simulink model "pulse_heating_official_spine_v04"  (R2025b)
settings: Solver=VariableStepAuto  StartTime=0.0  StopTime=0.25  RelTol=1e-3
PreLoadFcn:
  | addpath('C:\Users\ADMIN\Documents\MATLAB\Examples\R2025b\simscapeelectrical\BatteryThermalManagementExample');
  | addpath('C:\Users\ADMIN\Documents\MATLAB\Examples\R2025b\mcb\SIUnitsExample');
  | addpath('C:\Users\ADMIN\Documents\MATLAB\Examples\R2025b\simscapeelectrical\PMSMDriveThermalExample');
  | load_system('PMSMDriveThermal');
  | set_param('PMSMDriveThermal','SimscapeLogType','none','SimscapeLogSimulationStatistics','off');
  | set_param('PMSMDriveThermal','Dirty','off');
InitFcn:
  | % === M4-02A: Clean parameter matching (MO theory PI) ===
  | addpath('C:\Users\ADMIN\Documents\MATLAB\Examples\R2025b\simscapeelectrical\BatteryThermalManagementExample');
  | addpath('C:\Users\ADMIN\Documents\MATLAB\Examples\R2025b\mcb\SIUnitsExample');
  | addpath('C:\Users\ADMIN\Documents\MATLAB\Examples\R2025b\simscapeelectrical\PMSMDriveThermalExample');
  | load_system('PMSMDriveThermal');
  | PMSMDriveThermalData;
  | mcb_pmsm_foc_qep_f28379d_SIUnit_data;
  | clearvars('all');
  | 
  | % --- Construct clean pmsm struct from PMSMDriveThermal ---
  | pmsm = struct();
  | pmsm.Rs = Rs; pmsm.Ld = Ld; pmsm.Lq = Lq; pmsm.p = N; pmsm.FluxPM = PM;
  | pmsm.J = J; pmsm.B = 2.6369e-6; pmsm.I_rated = Imax;
  | pmsm.Ke = PM*N; pmsm.Kt = 1.5*N*PM; pmsm.N_max = 60*fnom/N;
  | pmsm.PositionOffset = 0; pmsm.QEPSlits = 1000;
  | 
  | inverter.V_dc = 70; dataType = 'double';
  | pmsm.N_base = inverter.V_dc / (sqrt(3)*PM*N*2*pi/60);
  | pmsm.T_rated = 1.5*N*PM*Imax;
  | 
  | % --- Timing (PMSMDriveThermal semantics) ---
  | Ts = 2e-6; fsw = 2e3; fc = fsw*10; Tsc = 1/fc;
  | T_pwm = 1/fsw; PWM_frequency = fsw; Ts_simulink = Tsc;
  | Ts_motor = Tsc; Ts_speed = 10*Tsc; Ts_inverter = Tsc;
  | 
  | % --- PI gains via mcb.calcFOCGains (MO theory) ---
  | motor = pmsm; motor.Rs = pmsm.Rs + inverter.R_board;
  | PI_params = mcb.calcFOCGains(motor, Tsc, Ts_speed, SpdLPFltCoeff=0.01);
  | PI_params.delay_Currents = int32(1);
  | PI_params.delay_Position = int32(1);
  | 
  | BatteryThermalManagementInitialization;
  | ambient = 263.15; coolantTemp = 263.15;
  | cellT_ini = ambient*ones(1,Ns*Np); cellT_ini4 = ambient*ones(1,Ns4*Np4);
  | Ns_total = 3*Ns + Ns4; Np_total = Np;
  | R_pack = Ns_total * R0_mat(3,2) / Np_total;
  | I_base_A = AH * Np_total; V_pack_nom = Ns_total * 3.3;
  | 
  | % === M4-01 generalized Reference / Platform contract ===
  | % Values are traceable engineering/platform defaults, not device ratings.
  | ReferenceConfig_ID = 'M4-01-REF-PLATFORM-v02';
  | ReferenceConfig_Source = 'OFFICIAL+ENGINEERING_DEFAULT';
  | ReferenceConfig_Scope = 'generalized_system_integration';
  | HVPath_R = 0.01;
  | DCLink_C = 470e-6;
  | DCLink_V0 = 0;
  | RMS_Window_s = 20/fsw;
  | IGBT_Ron_ref = 1e-3;
  | IGBT_Vf_ref = 1.2;
  | 
  | % Encoder/reference topology provides the static mechanical boundary.
  | OpenLoop_Vabc_Scale = 1;
model workspace (MAT data in the model file):
  control_status_v4d2_partial_duty_code = 6
  diagnostic_frequency_Hz = 50
  drive_status_v4d2_partial_current_code = 6
  kpi_status_v4d2_partial_numeric_code = 6
  kpi_value_unknown = nan
  limit_factor_unknown_code = 99
  limit_margin_unknown_value = nan
  limit_status_v4c_code = 5
  pulse_command_status_code = 6
  pulse_duty_percent = 50
  pulse_id_amplitude_A = 40
  pulse_iq_amplitude_A = 0
  pulse_mode_code = 4
  pulse_phase_delay_s = 0
undefined symbols (not defined in the file or in its folder): DiscIntNeverNeededParam, f_losses, Flowrate_vec, Isc_losses, losses_oc, losses_sc, N, PM, Rs
libraries: fl_lib x38, nesl_utility x35, ee_lib x12, mcbcontrolslib x5, mcbeeMathTransformLib x3, slpidlib x2, mcbhdlpositiondecoderlib x1, eePwmGeneratorTwoLevel x1
(part 3 of 4)

== system pulse_heating_official_spine_v04/PMSMDriveThermal_Inverter_And_Motor/Three-phase inverter ==
  G : Inport
  Demux : Demux  Outputs=6
  IGBT A(H) : ee_lib/Semiconductors & Converters/IGBT (Ideal, Switching)  port_option=ee.enum.controlport.ps  Vf=0.8 V  Ron=0.001 Ohm  Goff=1e-5 S  Vth=0.5 V  diode_param=2  diode_Vf=0.8 V  diode_Ron=0.001 Ohm  diode_Goff=1e-5 S  diode_C=5e-8 F  diode_iRM=-235 A  diode_iF=300 A  diode_idot=-50 A/us  diode_trr_param=1  diode_trr_factor=3  diode_trr=15 us  diode_Qrr=1.5e+3 s*uA  ice_specify=off  ice_priority=None  ice=0 A  ice_nominal_specify=off  ice_nominal_value=1  ice_nominal_unit=A  vce_specify=off  vce_priority=None  vce=0 V  vce_nominal_specify=off  vce_nominal_value=1  vce_nominal_unit=V  vge_specify=off  vge_priority=None  vge=0 V  vge_nominal_specify=off  vge_nominal_value=1  vge_nominal_unit=V  thermal_loss_option=ee.enum.converters.thermalLossOption.constantvalues  Von_data=[0, .1, .6, .8, 1, 1.3, 1.6, 2, 2.4; 0, .1, .7, 1, 1.2, 1.5, 1.9, 2.4, 2.8] V  Tj=[298.15, 398.15] K  Iout_data=[0, .1, 1, 5, 10, 20, 40, 70, 100] A  Eon_data=[0, .0024, .024, .12, .2, .48, 1.04, 2.16, 3.24; 0, .003, .03, .15, .25, .6, 1.3, 2.7, 4.05] * 1e-3 J  Eoff_data=[0, .0007, .0066, .033, .066, .17, .33, .83, 1.5; 0, .001, .01, .05, .1, .25, .5, 1.2, 2.2] * 1e-3 J  Eon_data_3D=[zeros(2, 9, 3)] J  Eoff_data_3D=[zeros(2, 9, 3)] J  Tj_loss=[298.15, 398.15] K  Iout_data_loss=[0, .1, 1, 5, 10, 20, 40, 70, 100] A  tabulateWithVce=false  Vce_loss=[0, 150, 300] V  Eon_scalar=22.86e-3 J  Eoff_scalar=17.14e-3 J  Voff=300 V  Iout_scalar=600 A  useCurrentFromPreviousCycle=false  useVoltageFromPreviousCycle=false  diodeModelType=ee.enum.converters.diodeModelType.pwl  diodeTableType=ee.enum.diode.tableType.IfMat  diode_ReverseIVType=ee.enum.diode.diodeReverseIV.constant  diode_IfMat=[.07, .12, .19, 1.75, 4.24, 7.32, 11.2; .16, .3, .72, 2.14, 4.02, 6.35, 9.12] A  diode_VfMat=[.9, 1.15, 1.25, 1.5, 1.75, 2.17, 2.6, 2.85; .58, .68, .75, 1.1, 1.38, 1.77, 2.27, 2.7] V  diode_TjVec=[25, 125] degC  diode_VfVec=[.5, .7, .9, 1.3, 1.7, 2.1, 2.5] V  diode_IfVec=[.1, .2, .5, 1, 2, 4, 7, 10] A  diode_IrMat=[1e-06, 2e-06, 5e-06, 1e-05, 2.5e-05, 5e-05, .0001; 2e-06, 5e-06, 1e-05, 4e-05, 8e-05, .0002, .0005] A  diode_VrMat=[10, 100, 200, 250, 300, 325, 350; 10, 70, 160, 220, 270, 300, 320] V  diode_VrVec=[10, 20, 40, 50, 70, 80, 100] V  diode_IrVec=[1e-06, 2e-06, 5e-06, 1e-05, 2e-05, 5e-05, .0001] A  diode_Vr=-600 V  diode_Ls=150 nH  diode_Erec=0.03 J  diode_rec_loss_model=ee.enum.diode.reverseRecoveryModel.fixed  diode_ErecVal=0 J  diode_scaleWithIandV=true  diode_ErecMat=zeros(2, 3) J  diode_TjrecVec=[298.15, 398.15] K  diode_IfrecVec=[.1, 1, 10] A  diode_IrecVal=10 A  diode_VrecVal=10 V  diode_tFilter=1 / 1000 / 100 s  separateThermalPortForDiode=false  thermal_network_parameterization=ee.enum.thermalNetworkTopology.external  Rth=[.08, .5] K/W  Rth_Cauer=[.08, .1, .5] K/W  Rth_Foster=[.08, .14, .22, .16] K/W  thermal_mass_parameterization=ee.enum.thermalNetwork.timeconstant  thermal_mass=[.01, .5] J/K  thermal_mass_Cauer=[.01, .1, .5] J/K  thermal_mass_Foster=[.001, .005, .05, .5] J/K  thermal_time_constant=[.001, .2] s  thermal_time_constant_Cauer=[.001, .1, .2] s  thermal_time_constant_Foster=[7e-05, .0007, .01, .08] s  thermal_mass_initial_temperatures=[25, 25] degC  thermal_mass_initial_temperatures_Cauer=[25, 25, 25] degC  junction_thermal_mass=0.01 J/K  Tvec_initial_Foster=[25, 25, 25, 25] degC  RthDiode=[.03, .2] K/W  RthCauerDiode=[.03, .1, .2] K/W  RthFosterDiode=[.03, .2] K/W  thermalMassDiode=[3, 25] J/K  thermalMassCauerDiode=[3, 10, 25] J/K  thermalMassFosterDiode=[33, 50] J/K  thermalTauDiode=[.1, 5] s  thermalTauCauerDiode=[.1, 1, 5] s  thermalTauFosterDiode=[1, 10] s  thermalMassInitTempDiode=[25, 25] degC  thermalMassInitTempCauerDiode=[25, 25, 25] degC  junctionthermalMassDiode=0.1 J/K  TVecInitialFosterDiode=[25, 25, 25, 25] degC  no_thermal_network=0  IGBT_junction_temperature_specify=off  IGBT_junction_temperature_priority=None  IGBT_junction_temperature=25 degC  IGBT_junction_temperature_nominal_specify=off  IGBT_junction_temperature_nominal_value=1  IGBT_junction_temperature_nominal_unit=degC  diode_junction_temperature_specify=off  diode_junction_temperature_priority=None  diode_junction_temperature=25 degC  diode_junction_temperature_nominal_specify=off  diode_junction_temperature_nominal_value=1  diode_junction_temperature_nominal_unit=degC  Qj_specify=off  Qj_priority=None  Qj=0 W  Qj_nominal_specify=off  Qj_nominal_value=1  Qj_nominal_unit=W  accumulatedSwitchingLosses_specify=off  accumulatedSwitchingLosses_priority=None  accumulatedSwitchingLosses=0 J
  IGBT A(L) : ee_lib/Semiconductors & Converters/IGBT (Ideal, Switching)  port_option=ee.enum.controlport.ps  Vf=0.8 V  Ron=0.001 Ohm  Goff=1e-5 S  Vth=0.5 V  diode_param=2  diode_Vf=0.8 V  diode_Ron=0.001 Ohm  diode_Goff=1e-5 S  diode_C=5e-8 F  diode_iRM=-235 A  diode_iF=300 A  diode_idot=-50 A/us  diode_trr_param=1  diode_trr_factor=3  diode_trr=15 us  diode_Qrr=1.5e+3 s*uA  ice_specify=off  ice_priority=None  ice=0 A  ice_nominal_specify=off  ice_nominal_value=1  ice_nominal_unit=A  vce_specify=off  vce_priority=None  vce=0 V  vce_nominal_specify=off  vce_nominal_value=1  vce_nominal_unit=V  vge_specify=off  vge_priority=None  vge=0 V  vge_nominal_specify=off  vge_nominal_value=1  vge_nominal_unit=V  thermal_loss_option=ee.enum.converters.thermalLossOption.constantvalues  Von_data=[0, .1, .6, .8, 1, 1.3, 1.6, 2, 2.4; 0, .1, .7, 1, 1.2, 1.5, 1.9, 2.4, 2.8] V  Tj=[298.15, 398.15] K  Iout_data=[0, .1, 1, 5, 10, 20, 40, 70, 100] A  Eon_data=[0, .0024, .024, .12, .2, .48, 1.04, 2.16, 3.24; 0, .003, .03, .15, .25, .6, 1.3, 2.7, 4.05] * 1e-3 J  Eoff_data=[0, .0007, .0066, .033, .066, .17, .33, .83, 1.5; 0, .001, .01, .05, .1, .25, .5, 1.2, 2.2] * 1e-3 J  Eon_data_3D=[zeros(2, 9, 3)] J  Eoff_data_3D=[zeros(2, 9, 3)] J  Tj_loss=[298.15, 398.15] K  Iout_data_loss=[0, .1, 1, 5, 10, 20, 40, 70, 100] A  tabulateWithVce=false  Vce_loss=[0, 150, 300] V  Eon_scalar=22.86e-3 J  Eoff_scalar=17.14e-3 J  Voff=300 V  Iout_scalar=600 A  useCurrentFromPreviousCycle=false  useVoltageFromPreviousCycle=false  diodeModelType=ee.enum.converters.diodeModelType.pwl  diodeTableType=ee.enum.diode.tableType.IfMat  diode_ReverseIVType=ee.enum.diode.diodeReverseIV.constant  diode_IfMat=[.07, .12, .19, 1.75, 4.24, 7.32, 11.2; .16, .3, .72, 2.14, 4.02, 6.35, 9.12] A  diode_VfMat=[.9, 1.15, 1.25, 1.5, 1.75, 2.17, 2.6, 2.85; .58, .68, .75, 1.1, 1.38, 1.77, 2.27, 2.7] V  diode_TjVec=[25, 125] degC  diode_VfVec=[.5, .7, .9, 1.3, 1.7, 2.1, 2.5] V  diode_IfVec=[.1, .2, .5, 1, 2, 4, 7, 10] A  diode_IrMat=[1e-06, 2e-06, 5e-06, 1e-05, 2.5e-05, 5e-05, .0001; 2e-06, 5e-06, 1e-05, 4e-05, 8e-05, .0002, .0005] A  diode_VrMat=[10, 100, 200, 250, 300, 325, 350; 10, 70, 160, 220, 270, 300, 320] V  diode_VrVec=[10, 20, 40, 50, 70, 80, 100] V  diode_IrVec=[1e-06, 2e-06, 5e-06, 1e-05, 2e-05, 5e-05, .0001] A  diode_Vr=-600 V  diode_Ls=150 nH  diode_Erec=0.03 J  diode_rec_loss_model=ee.enum.diode.reverseRecoveryModel.fixed  diode_ErecVal=0 J  diode_scaleWithIandV=true  diode_ErecMat=zeros(2, 3) J  diode_TjrecVec=[298.15, 398.15] K  diode_IfrecVec=[.1, 1, 10] A  diode_IrecVal=10 A  diode_VrecVal=10 V  diode_tFilter=1 / 1000 / 100 s  separateThermalPortForDiode=false  thermal_network_parameterization=ee.enum.thermalNetworkTopology.external  Rth=[.08, .5] K/W  Rth_Cauer=[.08, .1, .5] K/W  Rth_Foster=[.08, .14, .22, .16] K/W  thermal_mass_parameterization=ee.enum.thermalNetwork.timeconstant  thermal_mass=[.01, .5] J/K  thermal_mass_Cauer=[.01, .1, .5] J/K  thermal_mass_Foster=[.001, .005, .05, .5] J/K  thermal_time_constant=[.001, .2] s  thermal_time_constant_Cauer=[.001, .1, .2] s  thermal_time_constant_Foster=[7e-05, .0007, .01, .08] s  thermal_mass_initial_temperatures=[25, 25] degC  thermal_mass_initial_temperatures_Cauer=[25, 25, 25] degC  junction_thermal_mass=0.01 J/K  Tvec_initial_Foster=[25, 25, 25, 25] degC  RthDiode=[.03, .2] K/W  RthCauerDiode=[.03, .1, .2] K/W  RthFosterDiode=[.03, .2] K/W  thermalMassDiode=[3, 25] J/K  thermalMassCauerDiode=[3, 10, 25] J/K  thermalMassFosterDiode=[33, 50] J/K  thermalTauDiode=[.1, 5] s  thermalTauCauerDiode=[.1, 1, 5] s  thermalTauFosterDiode=[1, 10] s  thermalMassInitTempDiode=[25, 25] degC  thermalMassInitTempCauerDiode=[25, 25, 25] degC  junctionthermalMassDiode=0.1 J/K  TVecInitialFosterDiode=[25, 25, 25, 25] degC  no_thermal_network=0  IGBT_junction_temperature_specify=off  IGBT_junction_temperature_priority=None  IGBT_junction_temperature=25 degC  IGBT_junction_temperature_nominal_specify=off  IGBT_junction_temperature_nominal_value=1  IGBT_junction_temperature_nominal_unit=degC  diode_junction_temperature_specify=off  diode_junction_temperature_priority=None  diode_junction_temperature=25 degC  diode_junction_temperature_nominal_specify=off  diode_junction_temperature_nominal_value=1  diode_junction_temperature_nominal_unit=degC  Qj_specify=off  Qj_priority=None  Qj=0 W  Qj_nominal_specify=off  Qj_nominal_value=1  Qj_nominal_unit=W  accumulatedSwitchingLosses_specify=off  accumulatedSwitchingLosses_priority=None  accumulatedSwitchingLosses=0 J
  IGBT B(H) : ee_lib/Semiconductors & Converters/IGBT (Ideal, Switching)  port_option=ee.enum.controlport.ps  Vf=0.8 V  Ron=0.001 Ohm  Goff=1e-5 S  Vth=0.5 V  diode_param=2  diode_Vf=0.8 V  diode_Ron=0.001 Ohm  diode_Goff=1e-5 S  diode_C=5e-8 F  diode_iRM=-235 A  diode_iF=300 A  diode_idot=-50 A/us  diode_trr_param=1  diode_trr_factor=3  diode_trr=15 us  diode_Qrr=1.5e+3 s*uA  ice_specify=off  ice_priority=None  ice=0 A  ice_nominal_specify=off  ice_nominal_value=1  ice_nominal_unit=A  vce_specify=off  vce_priority=None  vce=0 V  vce_nominal_specify=off  vce_nominal_value=1  vce_nominal_unit=V  vge_specify=off  vge_priority=None  vge=0 V  vge_nominal_specify=off  vge_nominal_value=1  vge_nominal_unit=V  thermal_loss_option=ee.enum.converters.thermalLossOption.constantvalues  Von_data=[0, .1, .6, .8, 1, 1.3, 1.6, 2, 2.4; 0, .1, .7, 1, 1.2, 1.5, 1.9, 2.4, 2.8] V  Tj=[298.15, 398.15] K  Iout_data=[0, .1, 1, 5, 10, 20, 40, 70, 100] A  Eon_data=[0, .0024, .024, .12, .2, .48, 1.04, 2.16, 3.24; 0, .003, .03, .15, .25, .6, 1.3, 2.7, 4.05] * 1e-3 J  Eoff_data=[0, .0007, .0066, .033, .066, .17, .33, .83, 1.5; 0, .001, .01, .05, .1, .25, .5, 1.2, 2.2] * 1e-3 J  Eon_data_3D=[zeros(2, 9, 3)] J  Eoff_data_3D=[zeros(2, 9, 3)] J  Tj_loss=[298.15, 398.15] K  Iout_data_loss=[0, .1, 1, 5, 10, 20, 40, 70, 100] A  tabulateWithVce=false  Vce_loss=[0, 150, 300] V  Eon_scalar=22.86e-3 J  Eoff_scalar=17.14e-3 J  Voff=300 V  Iout_scalar=600 A  useCurrentFromPreviousCycle=false  useVoltageFromPreviousCycle=false  diodeModelType=ee.enum.converters.diodeModelType.pwl  diodeTableType=ee.enum.diode.tableType.IfMat  diode_ReverseIVType=ee.enum.diode.diodeReverseIV.constant  diode_IfMat=[.07, .12, .19, 1.75, 4.24, 7.32, 11.2; .16, .3, .72, 2.14, 4.02, 6.35, 9.12] A  diode_VfMat=[.9, 1.15, 1.25, 1.5, 1.75, 2.17, 2.6, 2.85; .58, .68, .75, 1.1, 1.38, 1.77, 2.27, 2.7] V  diode_TjVec=[25, 125] degC  diode_VfVec=[.5, .7, .9, 1.3, 1.7, 2.1, 2.5] V  diode_IfVec=[.1, .2, .5, 1, 2, 4, 7, 10] A  diode_IrMat=[1e-06, 2e-06, 5e-06, 1e-05, 2.5e-05, 5e-05, .0001; 2e-06, 5e-06, 1e-05, 4e-05, 8e-05, .0002, .0005] A  diode_VrMat=[10, 100, 200, 250, 300, 325, 350; 10, 70, 160, 220, 270, 300, 320] V  diode_VrVec=[10, 20, 40, 50, 70, 80, 100] V  diode_IrVec=[1e-06, 2e-06, 5e-06, 1e-05, 2e-05, 5e-05, .0001] A  diode_Vr=-600 V  diode_Ls=150 nH  diode_Erec=0.03 J  diode_rec_loss_model=ee.enum.diode.reverseRecoveryModel.fixed  diode_ErecVal=0 J  diode_scaleWithIandV=true  diode_ErecMat=zeros(2, 3) J  diode_TjrecVec=[298.15, 398.15] K  diode_IfrecVec=[.1, 1, 10] A  diode_IrecVal=10 A  diode_VrecVal=10 V  diode_tFilter=1 / 1000 / 100 s  separateThermalPortForDiode=false  thermal_network_parameterization=ee.enum.thermalNetworkTopology.external  Rth=[.08, .5] K/W  Rth_Cauer=[.08, .1, .5] K/W  Rth_Foster=[.08, .14, .22, .16] K/W  thermal_mass_parameterization=ee.enum.thermalNetwork.timeconstant  thermal_mass=[.01, .5] J/K  thermal_mass_Cauer=[.01, .1, .5] J/K  thermal_mass_Foster=[.001, .005, .05, .5] J/K  thermal_time_constant=[.001, .2] s  thermal_time_constant_Cauer=[.001, .1, .2] s  thermal_time_constant_Foster=[7e-05, .0007, .01, .08] s  thermal_mass_initial_temperatures=[25, 25] degC  thermal_mass_initial_temperatures_Cauer=[25, 25, 25] degC  junction_thermal_mass=0.01 J/K  Tvec_initial_Foster=[25, 25, 25, 25] degC  RthDiode=[.03, .2] K/W  RthCauerDiode=[.03, .1, .2] K/W  RthFosterDiode=[.03, .2] K/W  thermalMassDiode=[3, 25] J/K  thermalMassCauerDiode=[3, 10, 25] J/K  thermalMassFosterDiode=[33, 50] J/K  thermalTauDiode=[.1, 5] s  thermalTauCauerDiode=[.1, 1, 5] s  thermalTauFosterDiode=[1, 10] s  thermalMassInitTempDiode=[25, 25] degC  thermalMassInitTempCauerDiode=[25, 25, 25] degC  junctionthermalMassDiode=0.1 J/K  TVecInitialFosterDiode=[25, 25, 25, 25] degC  no_thermal_network=0  IGBT_junction_temperature_specify=off  IGBT_junction_temperature_priority=None  IGBT_junction_temperature=25 degC  IGBT_junction_temperature_nominal_specify=off  IGBT_junction_temperature_nominal_value=1  IGBT_junction_temperature_nominal_unit=degC  diode_junction_temperature_specify=off  diode_junction_temperature_priority=None  diode_junction_temperature=25 degC  diode_junction_temperature_nominal_specify=off  diode_junction_temperature_nominal_value=1  diode_junction_temperature_nominal_unit=degC  Qj_specify=off  Qj_priority=None  Qj=0 W  Qj_nominal_specify=off  Qj_nominal_value=1  Qj_nominal_unit=W  accumulatedSwitchingLosses_specify=off  accumulatedSwitchingLosses_priority=None  accumulatedSwitchingLosses=0 J
  IGBT B(L) : ee_lib/Semiconductors & Converters/IGBT (Ideal, Switching)  port_option=ee.enum.controlport.ps  Vf=0.8 V  Ron=0.001 Ohm  Goff=1e-5 S  Vth=0.5 V  diode_param=2  diode_Vf=0.8 V  diode_Ron=0.001 Ohm  diode_Goff=1e-5 S  diode_C=5e-8 F  diode_iRM=-235 A  diode_iF=300 A  diode_idot=-50 A/us  diode_trr_param=1  diode_trr_factor=3  diode_trr=15 us  diode_Qrr=1.5e+3 s*uA  ice_specify=off  ice_priority=None  ice=0 A  ice_nominal_specify=off  ice_nominal_value=1  ice_nominal_unit=A  vce_specify=off  vce_priority=None  vce=0 V  vce_nominal_specify=off  vce_nominal_value=1  vce_nominal_unit=V  vge_specify=off  vge_priority=None  vge=0 V  vge_nominal_specify=off  vge_nominal_value=1  vge_nominal_unit=V  thermal_loss_option=ee.enum.converters.thermalLossOption.constantvalues  Von_data=[0, .1, .6, .8, 1, 1.3, 1.6, 2, 2.4; 0, .1, .7, 1, 1.2, 1.5, 1.9, 2.4, 2.8] V  Tj=[298.15, 398.15] K  Iout_data=[0, .1, 1, 5, 10, 20, 40, 70, 100] A  Eon_data=[0, .0024, .024, .12, .2, .48, 1.04, 2.16, 3.24; 0, .003, .03, .15, .25, .6, 1.3, 2.7, 4.05] * 1e-3 J  Eoff_data=[0, .0007, .0066, .033, .066, .17, .33, .83, 1.5; 0, .001, .01, .05, .1, .25, .5, 1.2, 2.2] * 1e-3 J  Eon_data_3D=[zeros(2, 9, 3)] J  Eoff_data_3D=[zeros(2, 9, 3)] J  Tj_loss=[298.15, 398.15] K  Iout_data_loss=[0, .1, 1, 5, 10, 20, 40, 70, 100] A  tabulateWithVce=false  Vce_loss=[0, 150, 300] V  Eon_scalar=22.86e-3 J  Eoff_scalar=17.14e-3 J  Voff=300 V  Iout_scalar=600 A  useCurrentFromPreviousCycle=false  useVoltageFromPreviousCycle=false  diodeModelType=ee.enum.converters.diodeModelType.pwl  diodeTableType=ee.enum.diode.tableType.IfMat  diode_ReverseIVType=ee.enum.diode.diodeReverseIV.constant  diode_IfMat=[.07, .12, .19, 1.75, 4.24, 7.32, 11.2; .16, .3, .72, 2.14, 4.02, 6.35, 9.12] A  diode_VfMat=[.9, 1.15, 1.25, 1.5, 1.75, 2.17, 2.6, 2.85; .58, .68, .75, 1.1, 1.38, 1.77, 2.27, 2.7] V  diode_TjVec=[25, 125] degC  diode_VfVec=[.5, .7, .9, 1.3, 1.7, 2.1, 2.5] V  diode_IfVec=[.1, .2, .5, 1, 2, 4, 7, 10] A  diode_IrMat=[1e-06, 2e-06, 5e-06, 1e-05, 2.5e-05, 5e-05, .0001; 2e-06, 5e-06, 1e-05, 4e-05, 8e-05, .0002, .0005] A  diode_VrMat=[10, 100, 200, 250, 300, 325, 350; 10, 70, 160, 220, 270, 300, 320] V  diode_VrVec=[10, 20, 40, 50, 70, 80, 100] V  diode_IrVec=[1e-06, 2e-06, 5e-06, 1e-05, 2e-05, 5e-05, .0001] A  diode_Vr=-600 V  diode_Ls=150 nH  diode_Erec=0.03 J  diode_rec_loss_model=ee.enum.diode.reverseRecoveryModel.fixed  diode_ErecVal=0 J  diode_scaleWithIandV=true  diode_ErecMat=zeros(2, 3) J  diode_TjrecVec=[298.15, 398.15] K  diode_IfrecVec=[.1, 1, 10] A  diode_IrecVal=10 A  diode_VrecVal=10 V  diode_tFilter=1 / 1000 / 100 s  separateThermalPortForDiode=false  thermal_network_parameterization=ee.enum.thermalNetworkTopology.external  Rth=[.08, .5] K/W  Rth_Cauer=[.08, .1, .5] K/W  Rth_Foster=[.08, .14, .22, .16] K/W  thermal_mass_parameterization=ee.enum.thermalNetwork.timeconstant  thermal_mass=[.01, .5] J/K  thermal_mass_Cauer=[.01, .1, .5] J/K  thermal_mass_Foster=[.001, .005, .05, .5] J/K  thermal_time_constant=[.001, .2] s  thermal_time_constant_Cauer=[.001, .1, .2] s  thermal_time_constant_Foster=[7e-05, .0007, .01, .08] s  thermal_mass_initial_temperatures=[25, 25] degC  thermal_mass_initial_temperatures_Cauer=[25, 25, 25] degC  junction_thermal_mass=0.01 J/K  Tvec_initial_Foster=[25, 25, 25, 25] degC  RthDiode=[.03, .2] K/W  RthCauerDiode=[.03, .1, .2] K/W  RthFosterDiode=[.03, .2] K/W  thermalMassDiode=[3, 25] J/K  thermalMassCauerDiode=[3, 10, 25] J/K  thermalMassFosterDiode=[33, 50] J/K  thermalTauDiode=[.1, 5] s  thermalTauCauerDiode=[.1, 1, 5] s  thermalTauFosterDiode=[1, 10] s  thermalMassInitTempDiode=[25, 25] degC  thermalMassInitTempCauerDiode=[25, 25, 25] degC  junctionthermalMassDiode=0.1 J/K  TVecInitialFosterDiode=[25, 25, 25, 25] degC  no_thermal_network=0  IGBT_junction_temperature_specify=off  IGBT_junction_temperature_priority=None  IGBT_junction_temperature=25 degC  IGBT_junction_temperature_nominal_specify=off  IGBT_junction_temperature_nominal_value=1  IGBT_junction_temperature_nominal_unit=degC  diode_junction_temperature_specify=off  diode_junction_temperature_priority=None  diode_junction_temperature=25 degC  diode_junction_temperature_nominal_specify=off  diode_junction_temperature_nominal_value=1  diode_junction_temperature_nominal_unit=degC  Qj_specify=off  Qj_priority=None  Qj=0 W  Qj_nominal_specify=off  Qj_nominal_value=1  Qj_nominal_unit=W  accumulatedSwitchingLosses_specify=off  accumulatedSwitchingLosses_priority=None  accumulatedSwitchingLosses=0 J
  IGBT C(H) : ee_lib/Semiconductors & Converters/IGBT (Ideal, Switching)  port_option=ee.enum.controlport.ps  Vf=0.8 V  Ron=0.001 Ohm  Goff=1e-5 S  Vth=0.5 V  diode_param=2  diode_Vf=0.8 V  diode_Ron=0.001 Ohm  diode_Goff=1e-5 S  diode_C=5e-8 F  diode_iRM=-235 A  diode_iF=300 A  diode_idot=-50 A/us  diode_trr_param=1  diode_trr_factor=3  diode_trr=15 us  diode_Qrr=1.5e+3 s*uA  ice_specify=off  ice_priority=None  ice=0 A  ice_nominal_specify=off  ice_nominal_value=1  ice_nominal_unit=A  vce_specify=off  vce_priority=None  vce=0 V  vce_nominal_specify=off  vce_nominal_value=1  vce_nominal_unit=V  vge_specify=off  vge_priority=None  vge=0 V  vge_nominal_specify=off  vge_nominal_value=1  vge_nominal_unit=V  thermal_loss_option=ee.enum.converters.thermalLossOption.constantvalues  Von_data=[0, .1, .6, .8, 1, 1.3, 1.6, 2, 2.4; 0, .1, .7, 1, 1.2, 1.5, 1.9, 2.4, 2.8] V  Tj=[298.15, 398.15] K  Iout_data=[0, .1, 1, 5, 10, 20, 40, 70, 100] A  Eon_data=[0, .0024, .024, .12, .2, .48, 1.04, 2.16, 3.24; 0, .003, .03, .15, .25, .6, 1.3, 2.7, 4.05] * 1e-3 J  Eoff_data=[0, .0007, .0066, .033, .066, .17, .33, .83, 1.5; 0, .001, .01, .05, .1, .25, .5, 1.2, 2.2] * 1e-3 J  Eon_data_3D=[zeros(2, 9, 3)] J  Eoff_data_3D=[zeros(2, 9, 3)] J  Tj_loss=[298.15, 398.15] K  Iout_data_loss=[0, .1, 1, 5, 10, 20, 40, 70, 100] A  tabulateWithVce=false  Vce_loss=[0, 150, 300] V  Eon_scalar=22.86e-3 J  Eoff_scalar=17.14e-3 J  Voff=300 V  Iout_scalar=600 A  useCurrentFromPreviousCycle=false  useVoltageFromPreviousCycle=false  diodeModelType=ee.enum.converters.diodeModelType.pwl  diodeTableType=ee.enum.diode.tableType.IfMat  diode_ReverseIVType=ee.enum.diode.diodeReverseIV.constant  diode_IfMat=[.07, .12, .19, 1.75, 4.24, 7.32, 11.2; .16, .3, .72, 2.14, 4.02, 6.35, 9.12] A  diode_VfMat=[.9, 1.15, 1.25, 1.5, 1.75, 2.17, 2.6, 2.85; .58, .68, .75, 1.1, 1.38, 1.77, 2.27, 2.7] V  diode_TjVec=[25, 125] degC  diode_VfVec=[.5, .7, .9, 1.3, 1.7, 2.1, 2.5] V  diode_IfVec=[.1, .2, .5, 1, 2, 4, 7, 10] A  diode_IrMat=[1e-06, 2e-06, 5e-06, 1e-05, 2.5e-05, 5e-05, .0001; 2e-06, 5e-06, 1e-05, 4e-05, 8e-05, .0002, .0005] A  diode_VrMat=[10, 100, 200, 250, 300, 325, 350; 10, 70, 160, 220, 270, 300, 320] V  diode_VrVec=[10, 20, 40, 50, 70, 80, 100] V  diode_IrVec=[1e-06, 2e-06, 5e-06, 1e-05, 2e-05, 5e-05, .0001] A  diode_Vr=-600 V  diode_Ls=150 nH  diode_Erec=0.03 J  diode_rec_loss_model=ee.enum.diode.reverseRecoveryModel.fixed  diode_ErecVal=0 J  diode_scaleWithIandV=true  diode_ErecMat=zeros(2, 3) J  diode_TjrecVec=[298.15, 398.15] K  diode_IfrecVec=[.1, 1, 10] A  diode_IrecVal=10 A  diode_VrecVal=10 V  diode_tFilter=1 / 1000 / 100 s  separateThermalPortForDiode=false  thermal_network_parameterization=ee.enum.thermalNetworkTopology.external  Rth=[.08, .5] K/W  Rth_Cauer=[.08, .1, .5] K/W  Rth_Foster=[.08, .14, .22, .16] K/W  thermal_mass_parameterization=ee.enum.thermalNetwork.timeconstant  thermal_mass=[.01, .5] J/K  thermal_mass_Cauer=[.01, .1, .5] J/K  thermal_mass_Foster=[.001, .005, .05, .5] J/K  thermal_time_constant=[.001, .2] s  thermal_time_constant_Cauer=[.001, .1, .2] s  thermal_time_constant_Foster=[7e-05, .0007, .01, .08] s  thermal_mass_initial_temperatures=[25, 25] degC  thermal_mass_initial_temperatures_Cauer=[25, 25, 25] degC  junction_thermal_mass=0.01 J/K  Tvec_initial_Foster=[25, 25, 25, 25] degC  RthDiode=[.03, .2] K/W  RthCauerDiode=[.03, .1, .2] K/W  RthFosterDiode=[.03, .2] K/W  thermalMassDiode=[3, 25] J/K  thermalMassCauerDiode=[3, 10, 25] J/K  thermalMassFosterDiode=[33, 50] J/K  thermalTauDiode=[.1, 5] s  thermalTauCauerDiode=[.1, 1, 5] s  thermalTauFosterDiode=[1, 10] s  thermalMassInitTempDiode=[25, 25] degC  thermalMassInitTempCauerDiode=[25, 25, 25] degC  junctionthermalMassDiode=0.1 J/K  TVecInitialFosterDiode=[25, 25, 25, 25] degC  no_thermal_network=0  IGBT_junction_temperature_specify=off  IGBT_junction_temperature_priority=None  IGBT_junction_temperature=25 degC  IGBT_junction_temperature_nominal_specify=off  IGBT_junction_temperature_nominal_value=1  IGBT_junction_temperature_nominal_unit=degC  diode_junction_temperature_specify=off  diode_junction_temperature_priority=None  diode_junction_temperature=25 degC  diode_junction_temperature_nominal_specify=off  diode_junction_temperature_nominal_value=1  diode_junction_temperature_nominal_unit=degC  Qj_specify=off  Qj_priority=None  Qj=0 W  Qj_nominal_specify=off  Qj_nominal_value=1  Qj_nominal_unit=W  accumulatedSwitchingLosses_specify=off  accumulatedSwitchingLosses_priority=None  accumulatedSwitchingLosses=0 J
  IGBT C(L) : ee_lib/Semiconductors & Converters/IGBT (Ideal, Switching)  port_option=ee.enum.controlport.ps  Vf=0.8 V  Ron=0.001 Ohm  Goff=1e-5 S  Vth=0.5 V  diode_param=2  diode_Vf=0.8 V  diode_Ron=0.001 Ohm  diode_Goff=1e-5 S  diode_C=5e-8 F  diode_iRM=-235 A  diode_iF=300 A  diode_idot=-50 A/us  diode_trr_param=1  diode_trr_factor=3  diode_trr=15 us  diode_Qrr=1.5e+3 s*uA  ice_specify=off  ice_priority=None  ice=0 A  ice_nominal_specify=off  ice_nominal_value=1  ice_nominal_unit=A  vce_specify=off  vce_priority=None  vce=0 V  vce_nominal_specify=off  vce_nominal_value=1  vce_nominal_unit=V  vge_specify=off  vge_priority=None  vge=0 V  vge_nominal_specify=off  vge_nominal_value=1  vge_nominal_unit=V  thermal_loss_option=ee.enum.converters.thermalLossOption.constantvalues  Von_data=[0, .1, .6, .8, 1, 1.3, 1.6, 2, 2.4; 0, .1, .7, 1, 1.2, 1.5, 1.9, 2.4, 2.8] V  Tj=[298.15, 398.15] K  Iout_data=[0, .1, 1, 5, 10, 20, 40, 70, 100] A  Eon_data=[0, .0024, .024, .12, .2, .48, 1.04, 2.16, 3.24; 0, .003, .03, .15, .25, .6, 1.3, 2.7, 4.05] * 1e-3 J  Eoff_data=[0, .0007, .0066, .033, .066, .17, .33, .83, 1.5; 0, .001, .01, .05, .1, .25, .5, 1.2, 2.2] * 1e-3 J  Eon_data_3D=[zeros(2, 9, 3)] J  Eoff_data_3D=[zeros(2, 9, 3)] J  Tj_loss=[298.15, 398.15] K  Iout_data_loss=[0, .1, 1, 5, 10, 20, 40, 70, 100] A  tabulateWithVce=false  Vce_loss=[0, 150, 300] V  Eon_scalar=22.86e-3 J  Eoff_scalar=17.14e-3 J  Voff=300 V  Iout_scalar=600 A  useCurrentFromPreviousCycle=false  useVoltageFromPreviousCycle=false  diodeModelType=ee.enum.converters.diodeModelType.pwl  diodeTableType=ee.enum.diode.tableType.IfMat  diode_ReverseIVType=ee.enum.diode.diodeReverseIV.constant  diode_IfMat=[.07, .12, .19, 1.75, 4.24, 7.32, 11.2; .16, .3, .72, 2.14, 4.02, 6.35, 9.12] A  diode_VfMat=[.9, 1.15, 1.25, 1.5, 1.75, 2.17, 2.6, 2.85; .58, .68, .75, 1.1, 1.38, 1.77, 2.27, 2.7] V  diode_TjVec=[25, 125] degC  diode_VfVec=[.5, .7, .9, 1.3, 1.7, 2.1, 2.5] V  diode_IfVec=[.1, .2, .5, 1, 2, 4, 7, 10] A  diode_IrMat=[1e-06, 2e-06, 5e-06, 1e-05, 2.5e-05, 5e-05, .0001; 2e-06, 5e-06, 1e-05, 4e-05, 8e-05, .0002, .0005] A  diode_VrMat=[10, 100, 200, 250, 300, 325, 350; 10, 70, 160, 220, 270, 300, 320] V  diode_VrVec=[10, 20, 40, 50, 70, 80, 100] V  diode_IrVec=[1e-06, 2e-06, 5e-06, 1e-05, 2e-05, 5e-05, .0001] A  diode_Vr=-600 V  diode_Ls=150 nH  diode_Erec=0.03 J  diode_rec_loss_model=ee.enum.diode.reverseRecoveryModel.fixed  diode_ErecVal=0 J  diode_scaleWithIandV=true  diode_ErecMat=zeros(2, 3) J  diode_TjrecVec=[298.15, 398.15] K  diode_IfrecVec=[.1, 1, 10] A  diode_IrecVal=10 A  diode_VrecVal=10 V  diode_tFilter=1 / 1000 / 100 s  separateThermalPortForDiode=false  thermal_network_parameterization=ee.enum.thermalNetworkTopology.external  Rth=[.08, .5] K/W  Rth_Cauer=[.08, .1, .5] K/W  Rth_Foster=[.08, .14, .22, .16] K/W  thermal_mass_parameterization=ee.enum.thermalNetwork.timeconstant  thermal_mass=[.01, .5] J/K  thermal_mass_Cauer=[.01, .1, .5] J/K  thermal_mass_Foster=[.001, .005, .05, .5] J/K  thermal_time_constant=[.001, .2] s  thermal_time_constant_Cauer=[.001, .1, .2] s  thermal_time_constant_Foster=[7e-05, .0007, .01, .08] s  thermal_mass_initial_temperatures=[25, 25] degC  thermal_mass_initial_temperatures_Cauer=[25, 25, 25] degC  junction_thermal_mass=0.01 J/K  Tvec_initial_Foster=[25, 25, 25, 25] degC  RthDiode=[.03, .2] K/W  RthCauerDiode=[.03, .1, .2] K/W  RthFosterDiode=[.03, .2] K/W  thermalMassDiode=[3, 25] J/K  thermalMassCauerDiode=[3, 10, 25] J/K  thermalMassFosterDiode=[33, 50] J/K  thermalTauDiode=[.1, 5] s  thermalTauCauerDiode=[.1, 1, 5] s  thermalTauFosterDiode=[1, 10] s  thermalMassInitTempDiode=[25, 25] degC  thermalMassInitTempCauerDiode=[25, 25, 25] degC  junctionthermalMassDiode=0.1 J/K  TVecInitialFosterDiode=[25, 25, 25, 25] degC  no_thermal_network=0  IGBT_junction_temperature_specify=off  IGBT_junction_temperature_priority=None  IGBT_junction_temperature=25 degC  IGBT_junction_temperature_nominal_specify=off  IGBT_junction_temperature_nominal_value=1  IGBT_junction_temperature_nominal_unit=degC  diode_junction_temperature_specify=off  diode_junction_temperature_priority=None  diode_junction_temperature=25 degC  diode_junction_temperature_nominal_specify=off  diode_junction_temperature_nominal_value=1  diode_junction_temperature_nominal_unit=degC  Qj_specify=off  Qj_priority=None  Qj=0 W  Qj_nominal_specify=off  Qj_nominal_value=1  Qj_nominal_unit=W  accumulatedSwitchingLosses_specify=off  accumulatedSwitchingLosses_priority=None  accumulatedSwitchingLosses=0 J
  Phase Splitter : ee_lib/Connectors & References/Phase Splitter
  Simulink-PS G{1..6} (6 alike) : nesl_utility/Simulink-PS Converter  PhysicalDomain=network_engine_domain  SubClassName=ps_input  LeftPortType=input  RightPortType=output  PseudoPeriodic=off  Frequencies=[]  NoiseDistribution=none  NoiseParameters=[]  Unit=1  AffineConversion=off  FilteringAndDerivatives=zero  SimscapeFilterOrder=1  InputFilterTimeConstant=1e-6  UdotUserProvided=0
  ~ : PMIOPort  Tag=PMCPort  Side=Right
  + : PMIOPort  Tag=PMCPort  Port=2  Side=Left
  - : PMIOPort  Tag=PMCPort  Port=3  Side=Left
  wires:
  Demux/1 -> Simulink-PS G1/1
  G/1 -> Demux/1
  Demux/2 -> Simulink-PS G2/1
  Demux/3 -> Simulink-PS G3/1
  Demux/4 -> Simulink-PS G4/1
  Demux/5 -> Simulink-PS G5/1
  Demux/6 -> Simulink-PS G6/1
  connections:
  Simulink-PS G1/RConn1 -- IGBT A(H)/LConn1
  ~/RConn1 -- Phase Splitter/LConn1
  IGBT A(L)/LConn1 -- Simulink-PS G2/RConn1
  IGBT B(H)/LConn1 -- Simulink-PS G3/RConn1
  IGBT B(L)/LConn1 -- Simulink-PS G4/RConn1
  IGBT C(H)/LConn1 -- Simulink-PS G5/RConn1
  IGBT C(L)/LConn1 -- Simulink-PS G6/RConn1
  IGBT B(L)/RConn2 -- IGBT C(L)/RConn2 -- -/RConn1 -- IGBT A(L)/RConn2
  Phase Splitter/RConn1 -- IGBT A(H)/RConn2 -- IGBT A(L)/RConn1
  IGBT B(H)/RConn2 -- IGBT B(L)/RConn1 -- Phase Splitter/RConn2
  IGBT C(H)/RConn2 -- IGBT C(L)/RConn1 -- Phase Splitter/RConn3
  IGBT C(H)/RConn1 -- IGBT B(H)/RConn1 -- +/RConn1 -- IGBT A(H)/RConn1

== system pulse_heating_official_spine_v04/System_Audit/Battery_Envelope_Screening ==
  Compute_Battery_Limits_V4F : MATLAB Function  TreatAsAtomicUnit=on
  Compute_Lithium_Risk_V4F : MATLAB Function  TreatAsAtomicUnit=on
  Term_risk_flag : Terminator
  cellAH_param : Constant  Value=I_base_A
  tag scope: charge_limit_V4F=global, discharge_limit_V4F=global, safety_margin_V4F=global
  wires:
  Compute_Battery_Limits_V4F/1(charge_limit) -> [charge_limit_V4F]
  [charge_limit_V4F] -> Compute_Lithium_Risk_V4F/3(charge_limit)
  [T_min_V4F] -> Compute_Battery_Limits_V4F/1(T_min)
  Compute_Battery_Limits_V4F/2(discharge_limit) -> [discharge_limit_V4F]
  [T_min_V4F] -> Compute_Lithium_Risk_V4F/1(T_min)
  [SOC_1_V4F] -> Compute_Battery_Limits_V4F/2(SOC)
  [I_batt_meas] -> Compute_Lithium_Risk_V4F/2(I_pack)
  cellAH_param/1 -> Compute_Battery_Limits_V4F/3(cellAH)
  Compute_Lithium_Risk_V4F/2(safety_margin) -> [safety_margin_V4F]
  Compute_Lithium_Risk_V4F/1(risk_flag) -> Term_risk_flag/1

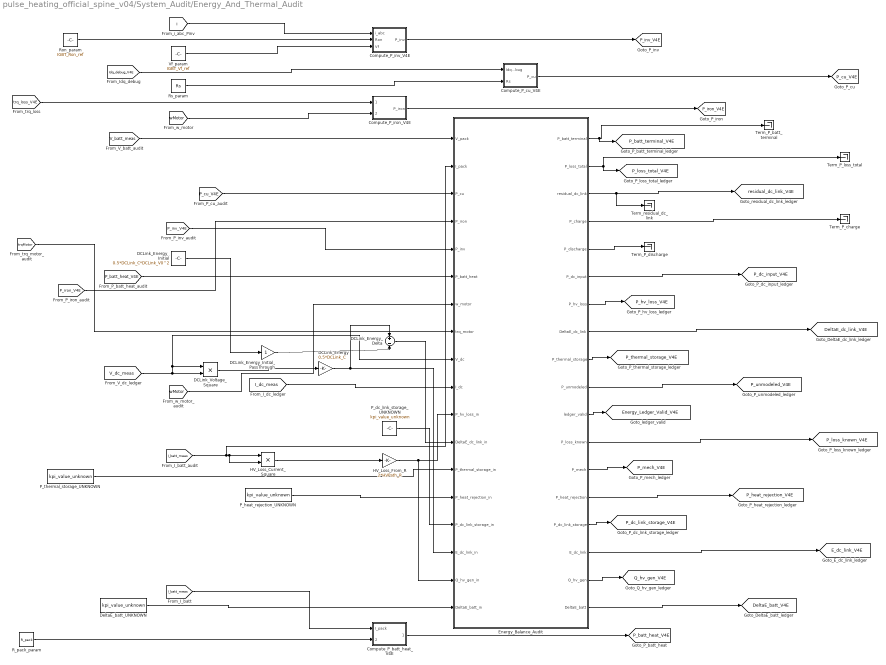
== system pulse_heating_official_spine_v04/System_Audit/Energy_And_Thermal_Audit ==
  Compute_P_batt_heat_V4E : MATLAB Function  TreatAsAtomicUnit=on
  Compute_P_cu_V4E : MATLAB Function  TreatAsAtomicUnit=on
  Compute_P_inv_V4E : MATLAB Function  TreatAsAtomicUnit=on
  Compute_P_iron_V4E : MATLAB Function  TreatAsAtomicUnit=on
  DCLink_Energy : Gain  Gain=0.5*DCLink_C
  DCLink_Energy_Delta : Sum  Inputs=+-
  DCLink_Energy_Initial : Constant  Value=0.5*DCLink_C*DCLink_V0^2
  DCLink_Energy_Initial_PassThrough : Gain
  DCLink_Voltage_Square : Product  Inputs=**
  DeltaE_batt_UNKNOWN : Constant  Value=kpi_value_unknown
  Energy_Balance_Audit : MATLAB Function  TreatAsAtomicUnit=on
  HV_Loss_Current_Square : Product  Inputs=**
  HV_Loss_From_R : Gain  Gain=2*HVPath_R
  P_dc_link_storage_UNKNOWN : Constant  Value=kpi_value_unknown
  P_heat_rejection_UNKNOWN : Constant  Value=kpi_value_unknown
  P_thermal_storage_UNKNOWN : Constant  Value=kpi_value_unknown
  R_pack_param : Constant  Value=R_pack
  Ron_param : Constant  Value=IGBT_Ron_ref
  Rs_param : Constant  Value=Rs
  Term_P_batt_terminal : Terminator
  Term_P_charge : Terminator
  Term_P_discharge : Terminator
  Term_P_loss_total : Terminator
  Term_residual_dc_link : Terminator
  Vf_param : Constant  Value=IGBT_Vf_ref
  tag scope: DeltaE_batt_V4E=global, DeltaE_dc_link_V4E=global, E_dc_link_V4E=global, Energy_Ledger_Valid_V4E=global, P_batt_heat_V4E=global, P_batt_terminal_V4E=global, P_cu_V4E=global, P_dc_input_V4E=global, P_dc_link_storage_V4E=global, P_heat_rejection_V4E=global, P_hv_loss_V4E=global, P_inv_V4E=global, P_iron_V4E=global, P_loss_known_V4E=global, P_loss_total_V4E=global, P_mech_V4E=global, P_thermal_storage_V4E=global, P_unmodeled_V4E=global, Q_hv_gen_V4E=global, residual_dc_link_V4E=global
  wires:
  DCLink_Energy_Delta/1 -> Energy_Balance_Audit/12(DeltaE_dc_link_in)
  DCLink_Energy_Initial_PassThrough/1 -> DCLink_Energy_Delta/2
  DCLink_Energy_Initial/1 -> DCLink_Energy_Initial_PassThrough/1
  DCLink_Energy/1 -> DCLink_Energy_Delta/1, Energy_Balance_Audit/16(E_dc_link_in)
  DCLink_Voltage_Square/1 -> DCLink_Energy/1
  HV_Loss_From_R/1 -> Energy_Balance_Audit/11(P_hv_loss_in), Energy_Balance_Audit/17(Q_hv_gen_in)
  HV_Loss_Current_Square/1 -> HV_Loss_From_R/1
  Compute_P_batt_heat_V4E/1(P_batt_heat) -> [P_batt_heat_V4E]
  Energy_Balance_Audit/12(P_loss_known) -> [P_loss_known_V4E]
  Energy_Balance_Audit/8(DeltaE_dc_link) -> [DeltaE_dc_link_V4E]
  Energy_Balance_Audit/7(P_hv_loss) -> [P_hv_loss_V4E]
  Energy_Balance_Audit/6(P_dc_input) -> [P_dc_input_V4E]
  Energy_Balance_Audit/13(P_mech) -> [P_mech_V4E]
  Energy_Balance_Audit/5(P_discharge) -> Term_P_discharge/1
  Energy_Balance_Audit/4(P_charge) -> Term_P_charge/1
  Energy_Balance_Audit/3(residual_dc_link) -> Term_residual_dc_link/1, [residual_dc_link_V4E]
  Energy_Balance_Audit/18(DeltaE_batt) -> [DeltaE_batt_V4E]
  Energy_Balance_Audit/2(P_loss_total) -> [P_loss_total_V4E], Term_P_loss_total/1
  Compute_P_iron_V4E/1(P_iron) -> [P_iron_V4E]
  Compute_P_inv_V4E/1(P_inv) -> [P_inv_V4E]
  R_pack_param/1 -> Compute_P_batt_heat_V4E/2(R_pack)
  DeltaE_batt_UNKNOWN/1 -> Energy_Balance_Audit/18(DeltaE_batt_in)
  Energy_Balance_Audit/16(E_dc_link) -> [E_dc_link_V4E]
  P_heat_rejection_UNKNOWN/1 -> Energy_Balance_Audit/14(P_heat_rejection_in)
  P_thermal_storage_UNKNOWN/1 -> Energy_Balance_Audit/13(P_thermal_storage_in)
  Energy_Balance_Audit/1(P_batt_terminal) -> [P_batt_terminal_V4E], Term_P_batt_terminal/1
  [I_dc_meas] -> Energy_Balance_Audit/10(I_dc)
  Energy_Balance_Audit/9(P_thermal_storage) -> [P_thermal_storage_V4E]
  [V_dc_meas] -> Energy_Balance_Audit/9(V_dc), DCLink_Voltage_Square/1, DCLink_Voltage_Square/2
  Energy_Balance_Audit/15(P_dc_link_storage) -> [P_dc_link_storage_V4E]
  [trqMotor] -> Energy_Balance_Audit/8(trq_motor)
  [I_batt_meas] -> Compute_P_batt_heat_V4E/1(I_pack)
  [P_batt_heat_V4E] -> Energy_Balance_Audit/6(P_batt_heat)
  [P_iron_V4E] -> Energy_Balance_Audit/4(P_iron)
  Energy_Balance_Audit/10(P_unmodeled) -> [P_unmodeled_V4E]
  [P_cu_V4E] -> Energy_Balance_Audit/3(P_cu)
  Energy_Balance_Audit/17(Q_hv_gen) -> [Q_hv_gen_V4E]
  [I_batt_meas] -> HV_Loss_Current_Square/1, HV_Loss_Current_Square/2, Energy_Balance_Audit/2(I_pack)
  [P_inv_V4E] -> Energy_Balance_Audit/5(P_inv)
  [V_batt_meas] -> Energy_Balance_Audit/1(V_pack)
  Compute_P_cu_V4E/1(P_cu) -> [P_cu_V4E]
  Rs_param/1 -> Compute_P_cu_V4E/2(Rs)
  [Idq_debug_V4E] -> Compute_P_cu_V4E/1(Idq_debug)
  [wMotor] -> Energy_Balance_Audit/7(w_motor)
  Vf_param/1 -> Compute_P_inv_V4E/3(Vf)
  Ron_param/1 -> Compute_P_inv_V4E/2(Ron)
  Energy_Balance_Audit/14(P_heat_rejection) -> [P_heat_rejection_V4E]
  [i] -> Compute_P_inv_V4E/1(i_abc)
  [trq_loss_V4E] -> Compute_P_iron_V4E/1(trq_loss)
  [wMotor] -> Compute_P_iron_V4E/2(w_motor)
  Energy_Balance_Audit/11(ledger_valid) -> [Energy_Ledger_Valid_V4E]
  P_dc_link_storage_UNKNOWN/1 -> Energy_Balance_Audit/15(P_dc_link_storage_in)

== system pulse_heating_official_spine_v04/System_Audit/RMS_And_Measurement_Audit ==
  Compute_I_rms_V4G : MATLAB Function  TreatAsAtomicUnit=on
  I_heat_equiv_UNKNOWN : Constant  Value=kpi_value_unknown
  RMS_Window_Clock : DigitalClock  SampleTime=1e-3
  RMS_Window_s_param : Constant  Value=RMS_Window_s
  tag scope: I_batt_rms_V4G=global, I_dc_rms_V4G=global, I_heat_equiv_rms_V4G=global, I_phase_rms_V4G=global, RMS_Window_Complete_V4G=global, RMS_Window_Elapsed_s_V4G=global, RMS_Window_s_V4G=global
  wires:
  [I_dc_meas] -> Compute_I_rms_V4G/2(I_dc)
  [I_batt_meas] -> Compute_I_rms_V4G/1(I_batt)
  RMS_Window_s_param/1 -> [RMS_Window_s_V4G], Compute_I_rms_V4G/6(window_s)
  [i] -> Compute_I_rms_V4G/3(i_phase)
  Compute_I_rms_V4G/2(I_dc_rms) -> [I_dc_rms_V4G]
  I_heat_equiv_UNKNOWN/1 -> Compute_I_rms_V4G/4(I_heat_equiv)
  RMS_Window_Clock/1 -> Compute_I_rms_V4G/5(t)
  Compute_I_rms_V4G/1(I_batt_rms) -> [I_batt_rms_V4G]
  Compute_I_rms_V4G/3(I_phase_rms) -> [I_phase_rms_V4G]
  Compute_I_rms_V4G/4(I_heat_equiv_rms) -> [I_heat_equiv_rms_V4G]
  Compute_I_rms_V4G/5(window_complete) -> [RMS_Window_Complete_V4G]
  Compute_I_rms_V4G/6(window_elapsed_s) -> [RMS_Window_Elapsed_s_V4G]

== system pulse_heating_official_spine_v04/BatteryThermalManagement_BatteryPack/Battery_pack/                        Flow Divide ==
  In1 : Inport
  Constant : Constant  Value=0.95
  Constant1 : Constant  Value=0.9
  Constant2 : Constant  Value=0.85
  Constant3 : Constant  Value=0.99
  Product{,1..3} (4 alike) : Product
  Out1 : Outport
  Out2 : Outport  Port=2
  Out3 : Outport  Port=3
  Out4 : Outport  Port=4
  wires:
  Product2/1 -> Out4/1
  Product3/1 -> Out1/1
  Constant2/1 -> Product2/2
  Product1/1 -> Out3/1
  Constant3/1 -> Product3/2
  In1/1 -> Product3/1, Product/1, Product1/1, Product2/1
  Product/1 -> Out2/1
  Constant/1 -> Product/2
  Constant1/1 -> Product1/2

== system pulse_heating_official_spine_v04/BatteryThermalManagement_BatteryPack/Coolant_control/    ==
  Coolant T : Inport
  Amb : Inport  Port=2
  Pack max T : Inport  Port=3
  Pack min T : Inport  Port=4
  Subtract1 : Sum  Inputs=+-
  T : Concatenate  NumInputs=3
  FlwT : Outport
  Temperature : Outport  Port=2
  wires:
  Amb/1 -> Subtract1/2
  Coolant T/1 -> T/1, Subtract1/1
  Pack max T/1 -> T/2
  Subtract1/1 -> FlwT/1
  Pack min T/1 -> T/3
  T/1 -> Temperature/1

== system pulse_heating_official_spine_v04/BatteryThermalManagement_BatteryPack/Coolant_control/FlwR estimation ==
  Amb : Inport
  T vec : Inport  Port=2
  Constant : Constant
  Constant1 : Constant  Value=0.2
  FlwR=f(cell_deltaT) : Subsystem
  FlwR=f(packT-ambientT) : Subsystem
  MinMax2 : MinMax  Function=max  ZeroCross=off
  MinMax3 : MinMax  ZeroCross=off
  MinMax5 : MinMax  Function=max  Inputs=2  ZeroCross=off
  max T : Outport
  min T : Outport  Port=2
  FlwR=f(T) : Outport  Port=3
  Step : Outport  Port=4
  wires:
  FlwR=f(packT-ambientT)/1(FlwR) -> MinMax5/2
  Amb/1 -> FlwR=f(packT-ambientT)/3(Ambient T)
  FlwR=f(cell_deltaT)/1(FlwR) -> MinMax5/1
  MinMax5/1 -> FlwR=f(T)/1
  T vec/1 -> MinMax2/1, MinMax3/1
  MinMax2/1 -> max T/1, FlwR=f(cell_deltaT)/1(Pack max T), FlwR=f(packT-ambientT)/1(Pack max T)
  MinMax3/1 -> FlwR=f(cell_deltaT)/2(Pack min T), min T/1
  Constant1/1 -> Step/1
  Constant/1 -> FlwR=f(cell_deltaT)/3(limit FlwR), FlwR=f(packT-ambientT)/2(FlwR limit)

== system pulse_heating_official_spine_v04/BatteryThermalManagement_BatteryPack/Coolant_control/SOC limits ==
  SOC vec : Inport
  " " : Concatenate
  MinMax : MinMax  Function=max  ZeroCross=off
  MinMax1 : MinMax  ZeroCross=off
  SOC min/max : Outport
  wires:
  MinMax/1 -> " "/1  "max"
  " "/1 -> SOC min/max/1
  SOC vec/1 -> MinMax/1, MinMax1/1
  MinMax1/1 -> " "/2  "min"

== system pulse_heating_official_spine_v04/BatteryThermalManagement_BatteryPack/Coolant_control/Subsystem1 ==
  frac : Inport
  step size : Inport  Port=2
  Flowrate vector : Inport  Port=3
  Flowrate-value : Subsystem
  FlwR limits : Subsystem
  Step generator : Subsystem
  FlwR_out : Outport
  Flowrate value : Outport  Port=2
  wires:
  FlwR limits/1(FlwR_out) -> Flowrate-value/1(FlwR), FlwR_out/1
  frac/1 -> Step generator/1(frac)
  Step generator/1(step output) -> FlwR limits/1(FlwR)
  Flowrate vector/1 -> Flowrate-value/2(Flowrate vector)
  Flowrate-value/1(Flowrate) -> Flowrate value/1
  step size/1 -> Step generator/2(step size)

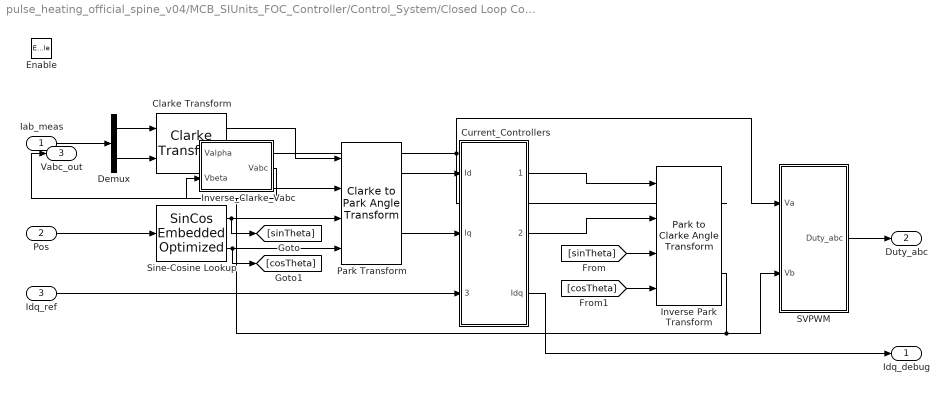
== system pulse_heating_official_spine_v04/MCB_SIUnits_FOC_Controller/Control_System/Closed Loop Control ==
  Iab_meas : Inport
  Pos : Inport  Port=2
  Idq_ref : Inport  Port=3
  Enable : EnablePort  StatesWhenEnabling=reset
  Clarke Transform : mcbeeMathTransformLib/Clarke Transform  VariantControl=Variant2  PowerInvariant=off  UseWithEmbedded=on  PhaseInput=Two inputs
      settings: LibrarySourceBlock=mcbcontrolslib/Clarke Transform
  Current_Controllers : Subsystem
  Demux : Demux  Outputs=2
  Inverse Park Transform : mcbeeMathTransformLib/Park to Clarke Angle Transform  AxisAlignment=Q-axis  UseWithEmbedded=on  PhaseInput=Two inputs  ThetaInput=Sine and Cosine electrical position  AngleInput=Per-unit  N_points=1024
      settings: LibrarySourceBlock=mcbcontrolslib/Inverse Park Transform
  Inverse_Clarke_Vabc : MATLAB Function  TreatAsAtomicUnit=on
  Park Transform : mcbeeMathTransformLib/Clarke to Park Angle Transform  AxisAlignment=Q-axis  UseWithEmbedded=on  PhaseInput=Two inputs  ThetaInput=Sine and Cosine electrical position  AngleInput=Per-unit  N_points=1024
      settings: LibrarySourceBlock=mcbcontrolslib/Park Transform
  SVPWM : Subsystem
  Sine-Cosine Lookup : mcbcontrolslib/SinCos Embedded Optimized  LabelModeActiveChoice=MCB_Sin  OptforProc=off  ApproximationMethod=None  UserApproxMethod=Lookup  ApproxStatus=None  InterpMethod=Linear point-slope  NumberOfDataPoints=16  NumberOfIterations=11  RemoveProtectionAgainstOutOfRangeInput=off  TableDataTypeStr=Inherit: Inherit via input  AngleInput=Radians  ThetaDataType=single  N_points=1024  DatatypeInput=Inherit from input  Datatype=Inherit: Same as input
  Idq_debug : Outport  VectorParamsAs1DForOutWhenUnconnected=off
  Duty_abc : Outport  Port=2  VectorParamsAs1DForOutWhenUnconnected=off
  Vabc_out : Outport  Port=3
  wires:
  SVPWM/1(Duty_abc) -> Duty_abc/1
  Current_Controllers/3(Idq) -> Idq_debug/1
  Current_Controllers/2(Vq_ref) -> Inverse Park Transform/2
  Current_Controllers/1(Vd_ref) -> Inverse Park Transform/1
  [sinTheta] -> Inverse Park Transform/3
  Demux/1 -> Clarke Transform/1
  Pos/1 -> Sine-Cosine Lookup/1
  Demux/2 -> Clarke Transform/2
  [cosTheta] -> Inverse Park Transform/4
  Clarke Transform/2 -> Park Transform/2
  Sine-Cosine Lookup/1 -> Park Transform/3, [sinTheta]
  Idq_ref/1 -> Current_Controllers/3(Ida_ref)
  Clarke Transform/1 -> Park Transform/1
  Sine-Cosine Lookup/2 -> [cosTheta], Park Transform/4
  Park Transform/1 -> Current_Controllers/1(Id)
  Park Transform/2 -> Current_Controllers/2(Iq)
  Iab_meas/1 -> Demux/1
  Inverse Park Transform/1 -> SVPWM/1(Va), Inverse_Clarke_Vabc/1(Valpha)
  Inverse Park Transform/2 -> Inverse_Clarke_Vabc/2(Vbeta), SVPWM/2(Vb)
  Inverse_Clarke_Vabc/1(Vabc) -> Vabc_out/1

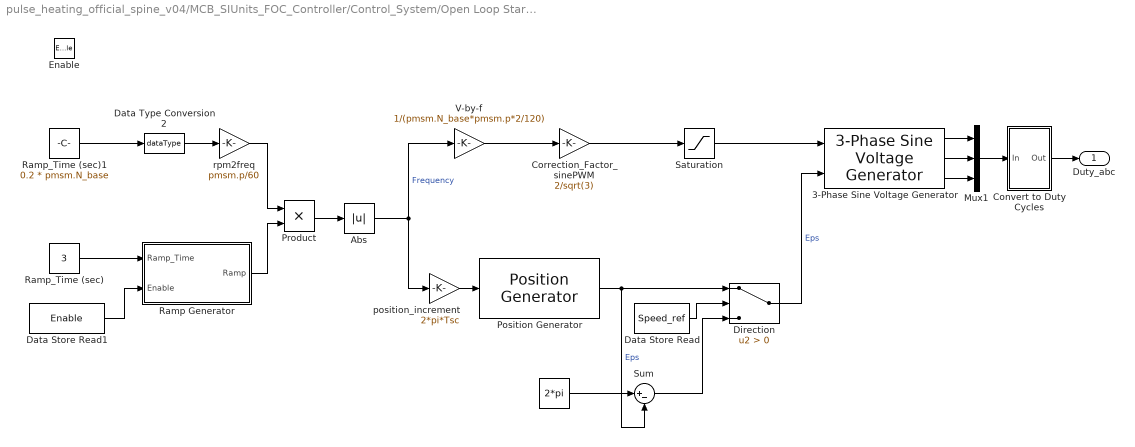
== system pulse_heating_official_spine_v04/MCB_SIUnits_FOC_Controller/Control_System/Open Loop Start-Up ==
  Enable : EnablePort  StatesWhenEnabling=reset
  " " : Constant  Value=2*pi  OutDataTypeStr=dataType  SampleTime=-1
  3-Phase Sine Voltage Generator : mcbcontrolslib/3-Phase Sine Voltage Generator  AngleInput=Radians  N_points=1024
  Abs : Abs  SaturateOnIntegerOverflow=off
  Convert to Duty Cycles : Subsystem
  Correction_Factor_sinePWM : Gain  Gain=2/sqrt(3)  RndMeth=Simplest  OutDataTypeStr=Inherit: Same as input
  Data Store Read : DataStoreRead  DataStoreName=Speed_ref  IndexOptions=Index vector (dialog)  Indices=1  OutputSizes=1
  Data Store Read1 : DataStoreRead  DataStoreName=Enable  IndexOptions=Index vector (dialog)  Indices=1  OutputSizes=1
  Data Type Conversion2 : DataTypeConversion  OutDataTypeStr=dataType  RndMeth=Simplest  SaturateOnIntegerOverflow=off
  Direction : Switch  Criteria=u2 > Threshold  OutDataTypeStr=dataType  RndMeth=Simplest  SaturateOnIntegerOverflow=off  InputSameDT=off
  Mux1 : Mux  Inputs=3
  Position Generator : mcbcontrolslib/Position Generator  AngleOutput=Radians  InitialThetaSource=Specify via dialog  ExternalReset=none  Offset=0
  Product : Product  RndMeth=Simplest  OutDataTypeStr=Inherit: Same as first input
  Ramp Generator : Subsystem
  Ramp_Time (sec) : Constant  Value=3  OutDataTypeStr=dataType  SampleTime=-1
  Ramp_Time (sec)1 : Constant  Value=0.2 * pmsm.N_base  OutDataTypeStr=dataType  SampleTime=-1
  Saturation : Saturate  UpperLimit=0.95  LowerLimit=0.15  RndMeth=Simplest
  Sum : Sum  Inputs=|+-  RndMeth=Simplest  OutDataTypeStr=Inherit: Same as first input
  V-by-f : Gain  Gain=1/(pmsm.N_base*pmsm.p*2/120)  RndMeth=Simplest  OutDataTypeStr=Inherit: Same as input
  position_increment : Gain  Gain=2*pi*Tsc  RndMeth=Simplest  OutDataTypeStr=Inherit: Same as input
  rpm2freq : Gain  Gain=pmsm.p/60  RndMeth=Simplest  OutDataTypeStr=Inherit: Same as input
  Duty_abc : Outport  VectorParamsAs1DForOutWhenUnconnected=off
  wires:
  Convert to Duty Cycles/1(Out) -> Duty_abc/1
  Mux1/1 -> Convert to Duty Cycles/1(In)
  Data Store Read/1 -> Direction/2
  Ramp_Time (sec)1/1 -> Data Type Conversion2/1
  Data Type Conversion2/1 -> rpm2freq/1
  3-Phase Sine Voltage Generator/2 -> Mux1/2
  Correction_Factor_sinePWM/1 -> Saturation/1
  Data Store Read1/1 -> Ramp Generator/2(Enable)
  rpm2freq/1 -> Product/1
  Product/1 -> Abs/1
  V-by-f/1 -> Correction_Factor_sinePWM/1
  position_increment/1 -> Position Generator/1
  Abs/1 -> V-by-f/1, position_increment/1  "Frequency"
  Sum/1 -> Direction/3
  " "/1 -> Sum/1
  Position Generator/1 -> Direction/1, Sum/2  "Eps"
  Ramp_Time (sec)/1 -> Ramp Generator/1(Ramp_Time)
  Ramp Generator/1(Ramp) -> Product/2
  Saturation/1 -> 3-Phase Sine Voltage Generator/1
  Direction/1 -> 3-Phase Sine Voltage Generator/2  "Eps"
  3-Phase Sine Voltage Generator/3 -> Mux1/3
  3-Phase Sine Voltage Generator/1 -> Mux1/1

== system pulse_heating_official_spine_v04/PMSMDriveThermal_Inverter_And_Motor/Scopes/losses ==
  idq : Inport
  w : Inport  Port=2
  Demux : Demux  Outputs=2
  MATLAB Function : MATLAB Function  TreatAsAtomicUnit=on
  tq_loss : Outport
  wires:
  Demux/2 -> MATLAB Function/2(i_q)
  Demux/1 -> MATLAB Function/1(i_d)
  idq/1 -> Demux/1
  MATLAB Function/1(trq_loss) -> tq_loss/1
  w/1 -> MATLAB Function/3(w)

== system pulse_heating_official_spine_v04/PMSMDriveThermal_Inverter_And_Motor/Thermal model/Sensing Temperature Rot ==
  PS-Simulink Converter : nesl_utility/PS-Simulink Converter  PhysicalDomain=network_engine_domain  SubClassName=ps_output  LeftPortType=input  RightPortType=output  PseudoPeriodic=off  Frequencies=[]  VectorFormat=1-D array  Unit=degC  AffineConversion=on
  Temperature Sensor : fl_lib/Thermal/Thermal Sensors/Temperature Sensor  temperature_measure=foundation.enum.MeasurementReference.difference
  ThRef : fl_lib/Thermal/Thermal Elements/Thermal Reference
  H : PMIOPort  Side=Left
  tag scope: TR=global
  wires:
  PS-Simulink Converter/1 -> [TR]
  connections:
  H/RConn1 -- Temperature Sensor/LConn1
  ThRef/LConn1 -- Temperature Sensor/RConn1
  Temperature Sensor/RConn2 -- PS-Simulink Converter/LConn1
